simulink model "VanDerPol"  (R2014b)
settings: Solver=ode45  StartTime=0.0  StopTime=100.0  FixedStep=1e-5  RelTol=1e-3
libraries: simulink x1
settings Model: Creator=Aluno  LastModifiedBy=Aluno

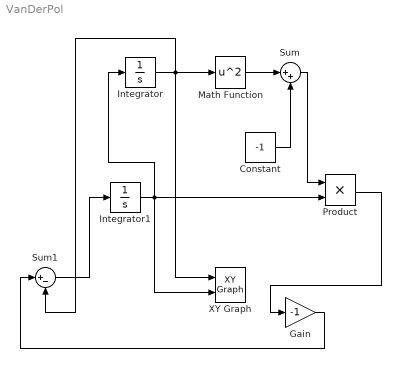
== system VanDerPol ==
  Constant : Constant  Value=-1
  Gain : Gain  Gain=-1
  Integrator : Integrator  InitialCondition=5
  Integrator1 : Integrator
  Math Function : Math  Operator=square  SampleTime=2  SaturateOnIntegerOverflow=on
  Product : Product
  Sum : Sum  Inputs=|++
  Sum1 : Sum  Inputs=|+-
  XY Graph : simulink/Sinks/XY Graph  xmin=-10  xmax=10  ymin=-10  ymax=10  st=-1
  wires:
  Integrator1/1 -> Product/2, XY Graph/2, Integrator/1
  Integrator/1 -> Math Function/1, Sum1/2, XY Graph/1
  Sum1/1 -> Integrator1/1
  Math Function/1 -> Sum/1
  Sum/1 -> Product/1
  Product/1 -> Gain/1
  Gain/1 -> Sum1/1
  Constant/1 -> Sum/2
